simulink model "C01A_DC_MotorEquation"  (R2024b)
settings: Solver=VariableStepAuto  StartTime=0.0  StopTime=0.2  RelTol=1e-3
undefined symbols (not defined in the file): b, J, Km, L, R, RadToRpm
settings Model: Creator=Davide  LastModifiedBy=Davide
settings DataIOCC: ReturnWorkspaceOutputs=off
settings OptimizationCC: ReuseModelBlockBuffer=off
settings RTWCC: GPUComputeCapability=3.5

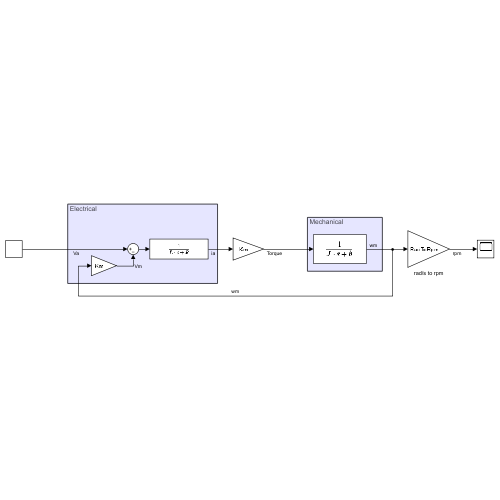
[thumbnail: Simulink's stored preview of the top-level diagram]
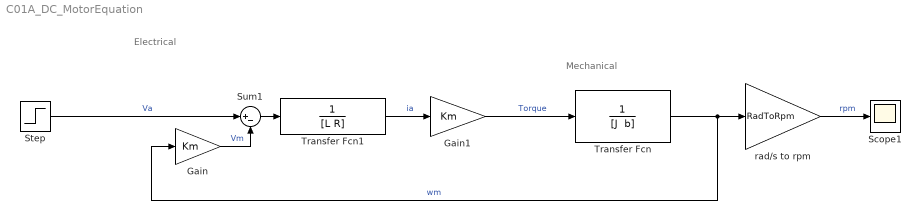
== system C01A_DC_MotorEquation ==
  note: Electrical
  note: Mechanical
  Gain : Gain  Gain=Km
  Gain1 : Gain  Gain=Km
  Scope1 : Scope
  Step : Step  Time=0  After=24  SampleTime=0
  Sum1 : Sum  Inputs=|+-
  Transfer Fcn : TransferFcn  Denominator="[J  b]"
  Transfer Fcn1 : TransferFcn  Denominator=[L R]
  rad/s to rpm : Gain  Gain=RadToRpm  SaturateOnIntegerOverflow=on  OutDataTypeStr=Inherit: Same as input  ParamDataTypeStr=Inherit: Same as input
  wires:
  rad/s to rpm/1 -> Scope1/1  "rpm"
  Transfer Fcn/1 -> rad/s to rpm/1, Gain/1  "wm"
  Transfer Fcn1/1 -> Gain1/1  "ia"
  Sum1/1 -> Transfer Fcn1/1
  Gain/1 -> Sum1/2  "Vm"
  Step/1 -> Sum1/1  "Va"
  Gain1/1 -> Transfer Fcn/1  "Torque"
